simulink model "control"  (R2014a)
settings: Solver=ode3  StartTime=0.0  StopTime=inf  FixedStep=Ts  RelTol=1e-3
InitFcn:
  | control_initfcn
StopFcn:
  | control_stopfcn
values from neighbouring files (symbols this model uses):
  Ts = 0.001    [Data_Analysis.m]    (also in control_initfcn.m = 0.01; estimation_initfcn.m)
undefined symbols (not defined in the file or in its folder): cobot1a, initPoseRightArm
libraries: sfbc_lib x2, rtai_devices x1
settings Model: SimulationMode=external  Creator=wirnshofer  LastModifiedBy=bschmidt
settings DataIOCC: SignalLoggingSaveFormat=ModelDataLogs
settings RTWCC: SystemTargetFile=prt.tlc  TemplateMakefile=prt.tmf  Description=Linux PREEMPT_RT Real-Time Target  ProcessScript=prt_make_rtw_hook
settings STFCustomTargetCC: TargetLangStandard=C99 (ISO)  CodeReplacementLibrary=GNU C99 extensions  ModelReferenceCompliant=off  ConcurrentExecutionCompliant=off  MatFileLogging=on  SystemTargetFile=prt.tlc
settings GRTTargetCC: TargetLangStandard=C99 (ISO)  CodeReplacementLibrary=GNU C99 extensions  ModelReferenceCompliant=off  ParMdlRefBuildCompliant=off  CompOptLevelCompliant=off  ConcurrentExecutionCompliant=off  CombineOutputUpdateFcns=off  CPPClassGenCompliant=off  GRTInterface=on  ExtMode=on  ExtModeMexArgs='cobot1b'

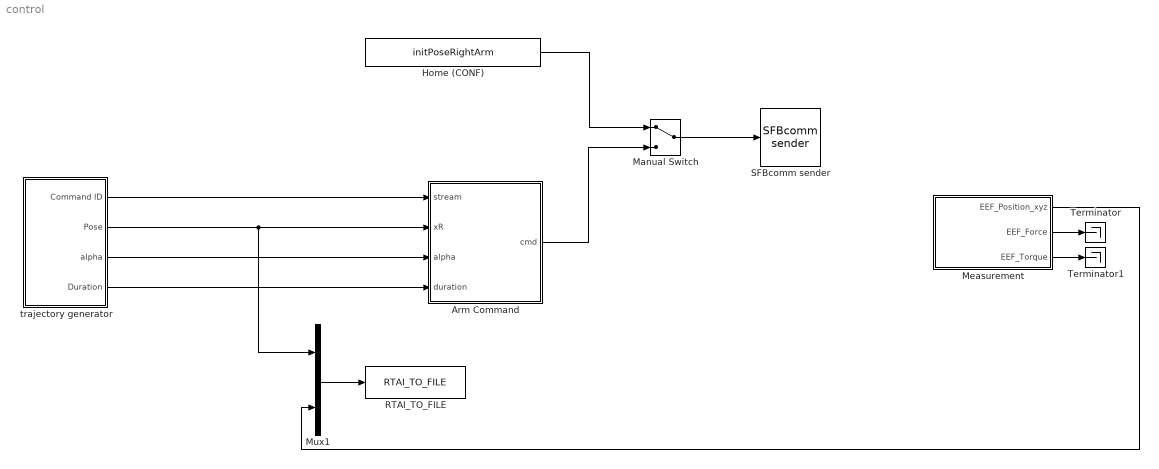
== system control ==
  Arm Command : Subsystem
  Home (CONF) : Constant  Value=initPoseRightArm  SampleTime=Ts
  Manual Switch : ManualSwitch
  Measurement : Subsystem
  Mux1 : Mux  Inputs=2
  RTAI_TO_FILE : rtai_devices/RTAI_TO_FILE  N=6  InType=double  FileName='follow.dat'  FpOutStr='%f '  TStartStop=[0 100]  T=Ts  Confirm=off  Cutoff=off
  SFBcomm sender : sfbc_lib/SFBcomm sender  localPort=8566  streamID=2  remoteSettings=cobot1a:8565  portNames=A  connectTimeout=200  sampleTime=-1
  Terminator : Terminator
  Terminator1 : Terminator
  trajectory generator : Subsystem
  wires:
  Manual Switch/1 -> SFBcomm sender/1
  Arm Command/1(cmd) -> Manual Switch/2
  Mux1/1 -> RTAI_TO_FILE/1
  Measurement/1(EEF_Position_xyz) -> Mux1/2
  Measurement/2(EEF_Force) -> Terminator/1
  Measurement/3(EEF_Torque) -> Terminator1/1
  Home (CONF)/1 -> Manual Switch/1
  trajectory generator/2(Pose) -> Arm Command/2(xR), Mux1/1
  trajectory generator/1(Command ID) -> Arm Command/1(stream)
  trajectory generator/3(alpha) -> Arm Command/3(alpha)
  trajectory generator/4(Duration) -> Arm Command/4(duration)

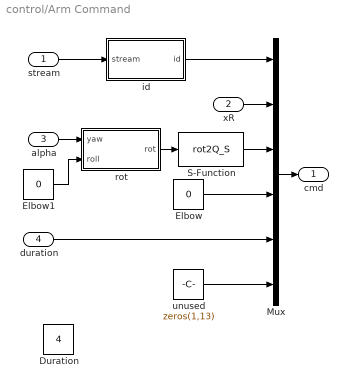
== system control/Arm Command ==
  stream : Inport
  xR : Inport  Port=2
  alpha : Inport  Port=3
  duration : Inport  Port=4
  Duration : Constant  Value=4
  Elbow : Constant  Value=0
  Elbow1 : Constant  Value=0
  Mux : Mux  Inputs=[1 3 4 1 1 13]
  S-Function : S-Function  FunctionName=rot2Q_S  EnableBusSupport=off
  id : MATLAB Function  TreatAsAtomicUnit=on
  rot : MATLAB Function  TreatAsAtomicUnit=on
  unused : Constant  Value=zeros(1,13)
  cmd : Outport
  wires:
  rot/1(rot) -> S-Function/1
  Elbow/1 -> Mux/4
  S-Function/1 -> Mux/3
  Elbow1/1 -> rot/2(roll)
  xR/1 -> Mux/2
  alpha/1 -> rot/1(yaw)
  Mux/1 -> cmd/1
  stream/1 -> id/1(stream)
  id/1(id) -> Mux/1
  unused/1 -> Mux/6
  duration/1 -> Mux/5

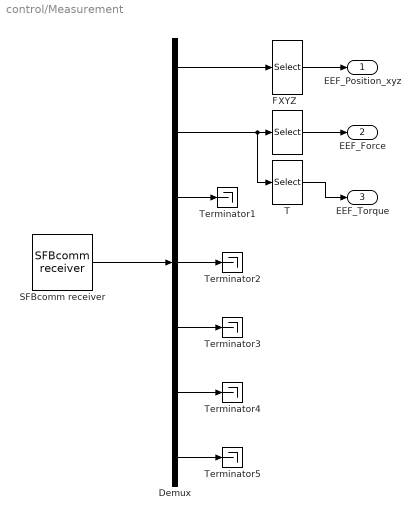
== system control/Measurement ==
  Demux : Demux  Outputs=[8 6 7 1 1 1 1]
  F : Selector  InputPortWidth=6  Indices=[1:3]
  SFBcomm receiver : sfbc_lib/SFBcomm receiver  localPort=8666  streamID=3  remoteSettings=cobot1a:8665  portNames=A  portWidths=25  outputLatency=off  outputIdleTime=off  connectTimeout=200  sampleTime=Ts
  T : Selector  InputPortWidth=6  Indices=[4:6]
  Terminator{1..5} (5 alike) : Terminator
  XYZ : Selector  InputPortWidth=8  Indices=[1:3]
  EEF_Position_xyz : Outport
  EEF_Force : Outport  Port=2
  EEF_Torque : Outport  Port=3
  wires:
  Demux/6 -> Terminator4/1
  Demux/2 -> T/1, F/1
  Demux/7 -> Terminator5/1
  Demux/5 -> Terminator3/1
  Demux/4 -> Terminator2/1
  XYZ/1 -> EEF_Position_xyz/1
  SFBcomm receiver/1 -> Demux/1
  Demux/1 -> XYZ/1
  F/1 -> EEF_Force/1
  T/1 -> EEF_Torque/1
  Demux/3 -> Terminator1/1

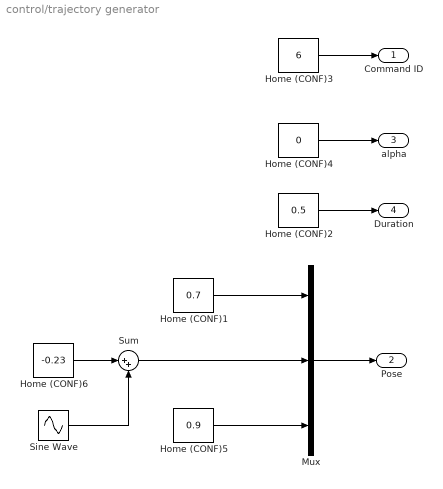
== system control/trajectory generator ==
  Home (CONF)1 : Constant  Value=0.7  SampleTime=Ts
  Home (CONF)2 : Constant  Value=0.5  SampleTime=Ts
  Home (CONF)3 : Constant  Value=6  SampleTime=Ts
  Home (CONF)4 : Constant  Value=0  SampleTime=Ts
  Home (CONF)5 : Constant  Value=0.9  SampleTime=Ts
  Home (CONF)6 : Constant  Value=-0.23  SampleTime=Ts
  Mux : Mux  Inputs=3
  Sine Wave : Sin  Amplitude=0.1  Frequency=0.1  SampleTime=0
  Sum : Sum  Inputs=|++
  Command ID : Outport
  Pose : Outport  Port=2
  alpha : Outport  Port=3
  Duration : Outport  Port=4
  wires:
  Home (CONF)3/1 -> Command ID/1
  Mux/1 -> Pose/1
  Home (CONF)4/1 -> alpha/1
  Home (CONF)2/1 -> Duration/1
  Home (CONF)1/1 -> Mux/1
  Home (CONF)5/1 -> Mux/3
  Sum/1 -> Mux/2
  Sine Wave/1 -> Sum/2
  Home (CONF)6/1 -> Sum/1

== matlab function control/Arm Command/id ==
  data: stream input; id output
function id = fcn(stream)
%#eml

if stream == 1
    id = 29;
else
    id = 6;
end

end

== matlab function control/Arm Command/rot ==
  data: yaw input; rot output; roll input
function rot = fcn(yaw,roll)
%#eml

rotZ = [ cos(yaw)  -sin(yaw) 0;
         sin(yaw)  cos(yaw)  0;
          0          0       1 ];
    
rotX = [ 1       0       0;
        0   cos(roll) -sin(roll);
        0   sin(roll)  cos(roll) ];
    
rot = rotZ * rotX;
